simulink model "simulator"  (R2019b)
settings: Solver=ode3  StartTime=0.0  StopTime=inf  FixedStep=0.5  RelTol=1e-3
InitFcn:
  | load('sim_buses');
undefined symbols (not defined in the file or in its folder): m, n
settings Model: OrderedModelArguments=off  Creator=Rafael.Casado  LastModifiedBy=paloma

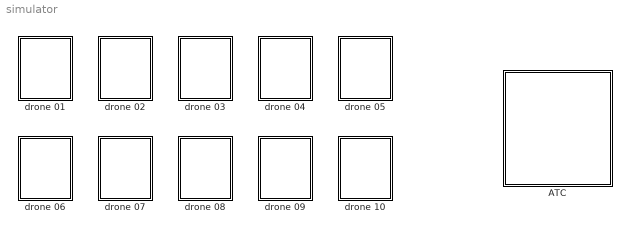
== system simulator ==
  ATC : Subsystem
      mask Display: image('$imagefile'); % Use "Edit Image" on toolstrip to change.
  drone 01 : Subsystem
      mask Display:
      | patch([50 -50 -50 50], [40 40 -60 -60], [1 1 1])
      | 
      | patch([8 -8 -8 8], [6 6 -6 -6], [0.7 0.7 0.7])
      | 
      | patch([ 8  8  28  28], [2 0 0 2], [0.5 0.5 0.5])
      | patch([-8 -8 -28 -28], [2 0 0 2], [0.5 0.5 0.5])
      | 
      | patch([ 30  46  30  14], [6 5 4 5], [1 0 0])
      | patch([-30 -46 -30 -14], [6 5 4 5], [1 0 0])
      | 
      | patch([ 28  28  32  32], [4 -2 -2 4], [0 0 0])
      | patch([-28 -28 -32 -32], [4 -2 -2 4], [0 0 0])
      | 
      | patch([ 8  12  11  7], [-6 -18 -18 -6], [0 0 0])
      | patch([-8 -12 -11 -7], [-6 -18 -18 -6], [0 0 0])
  drone 02 : Subsystem
      mask Display:
      | patch([50 -50 -50 50], [40 40 -60 -60], [1 1 1])
      | 
      | patch([8 -8 -8 8], [6 6 -6 -6], [0.7 0.7 0.7])
      | 
      | patch([ 8  8  28  28], [2 0 0 2], [0.5 0.5 0.5])
      | patch([-8 -8 -28 -28], [2 0 0 2], [0.5 0.5 0.5])
      | 
      | patch([ 30  46  30  14], [6 5 4 5], [1 0 0])
      | patch([-30 -46 -30 -14], [6 5 4 5], [1 0 0])
      | 
      | patch([ 28  28  32  32], [4 -2 -2 4], [0 0 0])
      | patch([-28 -28 -32 -32], [4 -2 -2 4], [0 0 0])
      | 
      | patch([ 8  12  11  7], [-6 -18 -18 -6], [0 0 0])
      | patch([-8 -12 -11 -7], [-6 -18 -18 -6], [0 0 0])
  drone 03 : Subsystem
      mask Display:
      | patch([50 -50 -50 50], [40 40 -60 -60], [1 1 1])
      | 
      | patch([8 -8 -8 8], [6 6 -6 -6], [0.7 0.7 0.7])
      | 
      | patch([ 8  8  28  28], [2 0 0 2], [0.5 0.5 0.5])
      | patch([-8 -8 -28 -28], [2 0 0 2], [0.5 0.5 0.5])
      | 
      | patch([ 30  46  30  14], [6 5 4 5], [1 0 0])
      | patch([-30 -46 -30 -14], [6 5 4 5], [1 0 0])
      | 
      | patch([ 28  28  32  32], [4 -2 -2 4], [0 0 0])
      | patch([-28 -28 -32 -32], [4 -2 -2 4], [0 0 0])
      | 
      | patch([ 8  12  11  7], [-6 -18 -18 -6], [0 0 0])
      | patch([-8 -12 -11 -7], [-6 -18 -18 -6], [0 0 0])
  drone 04 : Subsystem
      mask Display:
      | patch([50 -50 -50 50], [40 40 -60 -60], [1 1 1])
      | 
      | patch([8 -8 -8 8], [6 6 -6 -6], [0.7 0.7 0.7])
      | 
      | patch([ 8  8  28  28], [2 0 0 2], [0.5 0.5 0.5])
      | patch([-8 -8 -28 -28], [2 0 0 2], [0.5 0.5 0.5])
      | 
      | patch([ 30  46  30  14], [6 5 4 5], [1 0 0])
      | patch([-30 -46 -30 -14], [6 5 4 5], [1 0 0])
      | 
      | patch([ 28  28  32  32], [4 -2 -2 4], [0 0 0])
      | patch([-28 -28 -32 -32], [4 -2 -2 4], [0 0 0])
      | 
      | patch([ 8  12  11  7], [-6 -18 -18 -6], [0 0 0])
      | patch([-8 -12 -11 -7], [-6 -18 -18 -6], [0 0 0])
  drone 05 : Subsystem
      mask Display:
      | patch([50 -50 -50 50], [40 40 -60 -60], [1 1 1])
      | 
      | patch([8 -8 -8 8], [6 6 -6 -6], [0.7 0.7 0.7])
      | 
      | patch([ 8  8  28  28], [2 0 0 2], [0.5 0.5 0.5])
      | patch([-8 -8 -28 -28], [2 0 0 2], [0.5 0.5 0.5])
      | 
      | patch([ 30  46  30  14], [6 5 4 5], [1 0 0])
      | patch([-30 -46 -30 -14], [6 5 4 5], [1 0 0])
      | 
      | patch([ 28  28  32  32], [4 -2 -2 4], [0 0 0])
      | patch([-28 -28 -32 -32], [4 -2 -2 4], [0 0 0])
      | 
      | patch([ 8  12  11  7], [-6 -18 -18 -6], [0 0 0])
      | patch([-8 -12 -11 -7], [-6 -18 -18 -6], [0 0 0])
  drone 06 : Subsystem
      mask Display:
      | patch([50 -50 -50 50], [40 40 -60 -60], [1 1 1])
      | 
      | patch([8 -8 -8 8], [6 6 -6 -6], [0.7 0.7 0.7])
      | 
      | patch([ 8  8  28  28], [2 0 0 2], [0.5 0.5 0.5])
      | patch([-8 -8 -28 -28], [2 0 0 2], [0.5 0.5 0.5])
      | 
      | patch([ 30  46  30  14], [6 5 4 5], [1 0 0])
      | patch([-30 -46 -30 -14], [6 5 4 5], [1 0 0])
      | 
      | patch([ 28  28  32  32], [4 -2 -2 4], [0 0 0])
      | patch([-28 -28 -32 -32], [4 -2 -2 4], [0 0 0])
      | 
      | patch([ 8  12  11  7], [-6 -18 -18 -6], [0 0 0])
      | patch([-8 -12 -11 -7], [-6 -18 -18 -6], [0 0 0])
  drone 07 : Subsystem
      mask Display:
      | patch([50 -50 -50 50], [40 40 -60 -60], [1 1 1])
      | 
      | patch([8 -8 -8 8], [6 6 -6 -6], [0.7 0.7 0.7])
      | 
      | patch([ 8  8  28  28], [2 0 0 2], [0.5 0.5 0.5])
      | patch([-8 -8 -28 -28], [2 0 0 2], [0.5 0.5 0.5])
      | 
      | patch([ 30  46  30  14], [6 5 4 5], [1 0 0])
      | patch([-30 -46 -30 -14], [6 5 4 5], [1 0 0])
      | 
      | patch([ 28  28  32  32], [4 -2 -2 4], [0 0 0])
      | patch([-28 -28 -32 -32], [4 -2 -2 4], [0 0 0])
      | 
      | patch([ 8  12  11  7], [-6 -18 -18 -6], [0 0 0])
      | patch([-8 -12 -11 -7], [-6 -18 -18 -6], [0 0 0])
  drone 08 : Subsystem
      mask Display:
      | patch([50 -50 -50 50], [40 40 -60 -60], [1 1 1])
      | 
      | patch([8 -8 -8 8], [6 6 -6 -6], [0.7 0.7 0.7])
      | 
      | patch([ 8  8  28  28], [2 0 0 2], [0.5 0.5 0.5])
      | patch([-8 -8 -28 -28], [2 0 0 2], [0.5 0.5 0.5])
      | 
      | patch([ 30  46  30  14], [6 5 4 5], [1 0 0])
      | patch([-30 -46 -30 -14], [6 5 4 5], [1 0 0])
      | 
      | patch([ 28  28  32  32], [4 -2 -2 4], [0 0 0])
      | patch([-28 -28 -32 -32], [4 -2 -2 4], [0 0 0])
      | 
      | patch([ 8  12  11  7], [-6 -18 -18 -6], [0 0 0])
      | patch([-8 -12 -11 -7], [-6 -18 -18 -6], [0 0 0])
  drone 09 : Subsystem
      mask Display:
      | patch([50 -50 -50 50], [40 40 -60 -60], [1 1 1])
      | 
      | patch([8 -8 -8 8], [6 6 -6 -6], [0.7 0.7 0.7])
      | 
      | patch([ 8  8  28  28], [2 0 0 2], [0.5 0.5 0.5])
      | patch([-8 -8 -28 -28], [2 0 0 2], [0.5 0.5 0.5])
      | 
      | patch([ 30  46  30  14], [6 5 4 5], [1 0 0])
      | patch([-30 -46 -30 -14], [6 5 4 5], [1 0 0])
      | 
      | patch([ 28  28  32  32], [4 -2 -2 4], [0 0 0])
      | patch([-28 -28 -32 -32], [4 -2 -2 4], [0 0 0])
      | 
      | patch([ 8  12  11  7], [-6 -18 -18 -6], [0 0 0])
      | patch([-8 -12 -11 -7], [-6 -18 -18 -6], [0 0 0])
  drone 10 : Subsystem
      mask Display:
      | patch([50 -50 -50 50], [40 40 -60 -60], [1 1 1])
      | 
      | patch([8 -8 -8 8], [6 6 -6 -6], [0.7 0.7 0.7])
      | 
      | patch([ 8  8  28  28], [2 0 0 2], [0.5 0.5 0.5])
      | patch([-8 -8 -28 -28], [2 0 0 2], [0.5 0.5 0.5])
      | 
      | patch([ 30  46  30  14], [6 5 4 5], [1 0 0])
      | patch([-30 -46 -30 -14], [6 5 4 5], [1 0 0])
      | 
      | patch([ 28  28  32  32], [4 -2 -2 4], [0 0 0])
      | patch([-28 -28 -32 -32], [4 -2 -2 4], [0 0 0])
      | 
      | patch([ 8  12  11  7], [-6 -18 -18 -6], [0 0 0])
      | patch([-8 -12 -11 -7], [-6 -18 -18 -6], [0 0 0])

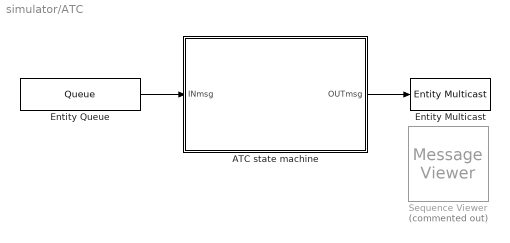
== system simulator/ATC ==
  ATC state machine : Stateflow chart  TreatAsAtomicUnit=on
  Entity Multicast : EntityMulticast  InputPortMessageModes=m  MulticastTag=msg
  Entity Queue : Queue  OutputPortMessageModes=m  Capacity=200  EntityArrivalSource=Multicast  MulticastTag=msg
  Sequence Viewer : MessageViewer  Commented=on  History=1000
  wires:
  Entity Queue/1 -> ATC state machine/1(INmsg)
  ATC state machine/1(OUTmsg) -> Entity Multicast/1

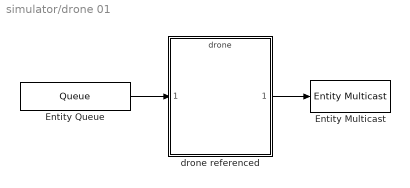
== system simulator/drone 01 ==
  Entity Multicast : EntityMulticast  InputPortMessageModes=m  MulticastTag=msg
  Entity Queue : Queue  OutputPortMessageModes=m  Capacity=105  EntityArrivalSource=Multicast  MulticastTag=msg
  drone referenced : ModelReference  InputPortMessageModes=m  OutputPortMessageModes=m  ModelNameDialog=drone  ParameterArgumentNames=UAVid  ParameterArgumentValues=1  UsingDefaultArgumentValue=0  SimulationMode=Normal  ModelReferenceVersion=1.1019
      mask Display:
      | patch([50 -50 -50 50], [40 40 -60 -60], [1 1 1])
      | 
      | patch([8 -8 -8 8], [6 6 -6 -6], [0.7 0.7 0.7])
      | 
      | patch([ 8  8  28  28], [2 0 0 2], [0.5 0.5 0.5])
      | patch([-8 -8 -28 -28], [2 0 0 2], [0.5 0.5 0.5])
      | 
      | patch([ 30  46  30  14], [6 5 4 5], [1 0 0])
      | patch([-30 -46 -30 -14], [6 5 4 5], [1 0 0])
      | 
      | patch([ 28  28  32  32], [4 -2 -2 4], [0 0 0])
      | patch([-28 -28 -32 -32], [4 -2 -2 4], [0 0 0])
      | 
      | patch([ 8  12  11  7], [-6 -18 -18 -6], [0 0 0])
      | patch([-8 -12 -11 -7], [-6 -18 -18 -6], [0 0 0])
  wires:
  drone referenced/1 -> Entity Multicast/1
  Entity Queue/1 -> drone referenced/1

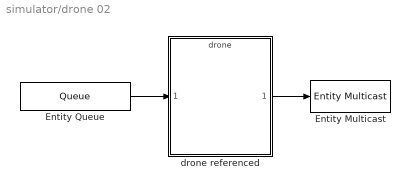
== system simulator/drone 02 ==
  Entity Multicast : EntityMulticast  InputPortMessageModes=m  MulticastTag=msg
  Entity Queue : Queue  OutputPortMessageModes=m  Capacity=105  EntityArrivalSource=Multicast  MulticastTag=msg
  drone referenced : ModelReference  InputPortMessageModes=m  OutputPortMessageModes=m  ModelNameDialog=drone  ParameterArgumentNames=UAVid  ParameterArgumentValues=2  UsingDefaultArgumentValue=0  SimulationMode=Normal  ModelReferenceVersion=1.1019
      mask Display:
      | patch([50 -50 -50 50], [40 40 -60 -60], [1 1 1])
      | 
      | patch([8 -8 -8 8], [6 6 -6 -6], [0.7 0.7 0.7])
      | 
      | patch([ 8  8  28  28], [2 0 0 2], [0.5 0.5 0.5])
      | patch([-8 -8 -28 -28], [2 0 0 2], [0.5 0.5 0.5])
      | 
      | patch([ 30  46  30  14], [6 5 4 5], [1 0 0])
      | patch([-30 -46 -30 -14], [6 5 4 5], [1 0 0])
      | 
      | patch([ 28  28  32  32], [4 -2 -2 4], [0 0 0])
      | patch([-28 -28 -32 -32], [4 -2 -2 4], [0 0 0])
      | 
      | patch([ 8  12  11  7], [-6 -18 -18 -6], [0 0 0])
      | patch([-8 -12 -11 -7], [-6 -18 -18 -6], [0 0 0])
  wires:
  drone referenced/1 -> Entity Multicast/1
  Entity Queue/1 -> drone referenced/1

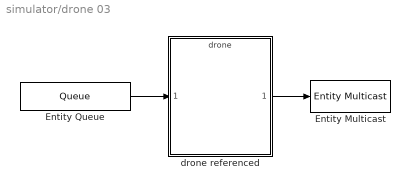
== system simulator/drone 03 ==
  Entity Multicast : EntityMulticast  InputPortMessageModes=m  MulticastTag=msg
  Entity Queue : Queue  OutputPortMessageModes=m  Capacity=105  EntityArrivalSource=Multicast  MulticastTag=msg
  drone referenced : ModelReference  InputPortMessageModes=m  OutputPortMessageModes=m  ModelNameDialog=drone  ParameterArgumentNames=UAVid  ParameterArgumentValues=3  UsingDefaultArgumentValue=0  SimulationMode=Normal  ModelReferenceVersion=1.1019
      mask Display:
      | patch([50 -50 -50 50], [40 40 -60 -60], [1 1 1])
      | 
      | patch([8 -8 -8 8], [6 6 -6 -6], [0.7 0.7 0.7])
      | 
      | patch([ 8  8  28  28], [2 0 0 2], [0.5 0.5 0.5])
      | patch([-8 -8 -28 -28], [2 0 0 2], [0.5 0.5 0.5])
      | 
      | patch([ 30  46  30  14], [6 5 4 5], [1 0 0])
      | patch([-30 -46 -30 -14], [6 5 4 5], [1 0 0])
      | 
      | patch([ 28  28  32  32], [4 -2 -2 4], [0 0 0])
      | patch([-28 -28 -32 -32], [4 -2 -2 4], [0 0 0])
      | 
      | patch([ 8  12  11  7], [-6 -18 -18 -6], [0 0 0])
      | patch([-8 -12 -11 -7], [-6 -18 -18 -6], [0 0 0])
  wires:
  drone referenced/1 -> Entity Multicast/1
  Entity Queue/1 -> drone referenced/1

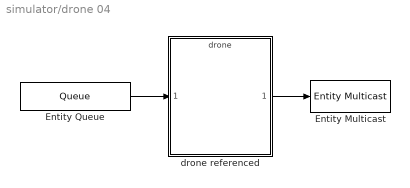
== system simulator/drone 04 ==
  Entity Multicast : EntityMulticast  InputPortMessageModes=m  MulticastTag=msg
  Entity Queue : Queue  OutputPortMessageModes=m  Capacity=105  EntityArrivalSource=Multicast  MulticastTag=msg
  drone referenced : ModelReference  InputPortMessageModes=m  OutputPortMessageModes=m  ModelNameDialog=drone  ParameterArgumentNames=UAVid  ParameterArgumentValues=4  UsingDefaultArgumentValue=0  SimulationMode=Normal  ModelReferenceVersion=1.1019
      mask Display:
      | patch([50 -50 -50 50], [40 40 -60 -60], [1 1 1])
      | 
      | patch([8 -8 -8 8], [6 6 -6 -6], [0.7 0.7 0.7])
      | 
      | patch([ 8  8  28  28], [2 0 0 2], [0.5 0.5 0.5])
      | patch([-8 -8 -28 -28], [2 0 0 2], [0.5 0.5 0.5])
      | 
      | patch([ 30  46  30  14], [6 5 4 5], [1 0 0])
      | patch([-30 -46 -30 -14], [6 5 4 5], [1 0 0])
      | 
      | patch([ 28  28  32  32], [4 -2 -2 4], [0 0 0])
      | patch([-28 -28 -32 -32], [4 -2 -2 4], [0 0 0])
      | 
      | patch([ 8  12  11  7], [-6 -18 -18 -6], [0 0 0])
      | patch([-8 -12 -11 -7], [-6 -18 -18 -6], [0 0 0])
  wires:
  drone referenced/1 -> Entity Multicast/1
  Entity Queue/1 -> drone referenced/1

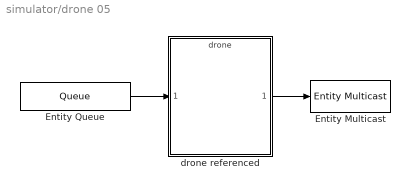
== system simulator/drone 05 ==
  Entity Multicast : EntityMulticast  InputPortMessageModes=m  MulticastTag=msg
  Entity Queue : Queue  OutputPortMessageModes=m  Capacity=105  EntityArrivalSource=Multicast  MulticastTag=msg
  drone referenced : ModelReference  InputPortMessageModes=m  OutputPortMessageModes=m  ModelNameDialog=drone  ParameterArgumentNames=UAVid  ParameterArgumentValues=5  UsingDefaultArgumentValue=0  SimulationMode=Normal  ModelReferenceVersion=1.1019
      mask Display:
      | patch([50 -50 -50 50], [40 40 -60 -60], [1 1 1])
      | 
      | patch([8 -8 -8 8], [6 6 -6 -6], [0.7 0.7 0.7])
      | 
      | patch([ 8  8  28  28], [2 0 0 2], [0.5 0.5 0.5])
      | patch([-8 -8 -28 -28], [2 0 0 2], [0.5 0.5 0.5])
      | 
      | patch([ 30  46  30  14], [6 5 4 5], [1 0 0])
      | patch([-30 -46 -30 -14], [6 5 4 5], [1 0 0])
      | 
      | patch([ 28  28  32  32], [4 -2 -2 4], [0 0 0])
      | patch([-28 -28 -32 -32], [4 -2 -2 4], [0 0 0])
      | 
      | patch([ 8  12  11  7], [-6 -18 -18 -6], [0 0 0])
      | patch([-8 -12 -11 -7], [-6 -18 -18 -6], [0 0 0])
  wires:
  drone referenced/1 -> Entity Multicast/1
  Entity Queue/1 -> drone referenced/1

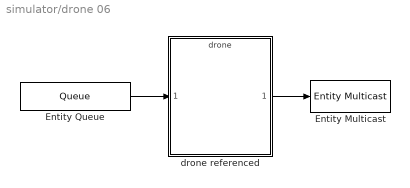
== system simulator/drone 06 ==
  Entity Multicast : EntityMulticast  InputPortMessageModes=m  MulticastTag=msg
  Entity Queue : Queue  OutputPortMessageModes=m  Capacity=105  EntityArrivalSource=Multicast  MulticastTag=msg
  drone referenced : ModelReference  InputPortMessageModes=m  OutputPortMessageModes=m  ModelNameDialog=drone  ParameterArgumentNames=UAVid  ParameterArgumentValues=6  UsingDefaultArgumentValue=0  SimulationMode=Normal  ModelReferenceVersion=1.1019
      mask Display:
      | patch([50 -50 -50 50], [40 40 -60 -60], [1 1 1])
      | 
      | patch([8 -8 -8 8], [6 6 -6 -6], [0.7 0.7 0.7])
      | 
      | patch([ 8  8  28  28], [2 0 0 2], [0.5 0.5 0.5])
      | patch([-8 -8 -28 -28], [2 0 0 2], [0.5 0.5 0.5])
      | 
      | patch([ 30  46  30  14], [6 5 4 5], [1 0 0])
      | patch([-30 -46 -30 -14], [6 5 4 5], [1 0 0])
      | 
      | patch([ 28  28  32  32], [4 -2 -2 4], [0 0 0])
      | patch([-28 -28 -32 -32], [4 -2 -2 4], [0 0 0])
      | 
      | patch([ 8  12  11  7], [-6 -18 -18 -6], [0 0 0])
      | patch([-8 -12 -11 -7], [-6 -18 -18 -6], [0 0 0])
  wires:
  drone referenced/1 -> Entity Multicast/1
  Entity Queue/1 -> drone referenced/1

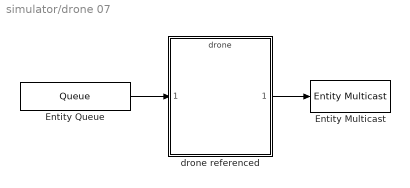
== system simulator/drone 07 ==
  Entity Multicast : EntityMulticast  InputPortMessageModes=m  MulticastTag=msg
  Entity Queue : Queue  OutputPortMessageModes=m  Capacity=105  EntityArrivalSource=Multicast  MulticastTag=msg
  drone referenced : ModelReference  InputPortMessageModes=m  OutputPortMessageModes=m  ModelNameDialog=drone  ParameterArgumentNames=UAVid  ParameterArgumentValues=7  UsingDefaultArgumentValue=0  SimulationMode=Normal  ModelReferenceVersion=1.1019
      mask Display:
      | patch([50 -50 -50 50], [40 40 -60 -60], [1 1 1])
      | 
      | patch([8 -8 -8 8], [6 6 -6 -6], [0.7 0.7 0.7])
      | 
      | patch([ 8  8  28  28], [2 0 0 2], [0.5 0.5 0.5])
      | patch([-8 -8 -28 -28], [2 0 0 2], [0.5 0.5 0.5])
      | 
      | patch([ 30  46  30  14], [6 5 4 5], [1 0 0])
      | patch([-30 -46 -30 -14], [6 5 4 5], [1 0 0])
      | 
      | patch([ 28  28  32  32], [4 -2 -2 4], [0 0 0])
      | patch([-28 -28 -32 -32], [4 -2 -2 4], [0 0 0])
      | 
      | patch([ 8  12  11  7], [-6 -18 -18 -6], [0 0 0])
      | patch([-8 -12 -11 -7], [-6 -18 -18 -6], [0 0 0])
  wires:
  drone referenced/1 -> Entity Multicast/1
  Entity Queue/1 -> drone referenced/1

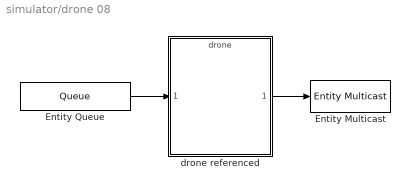
== system simulator/drone 08 ==
  Entity Multicast : EntityMulticast  InputPortMessageModes=m  MulticastTag=msg
  Entity Queue : Queue  OutputPortMessageModes=m  Capacity=105  EntityArrivalSource=Multicast  MulticastTag=msg
  drone referenced : ModelReference  InputPortMessageModes=m  OutputPortMessageModes=m  ModelNameDialog=drone  ParameterArgumentNames=UAVid  ParameterArgumentValues=8  UsingDefaultArgumentValue=0  SimulationMode=Normal  ModelReferenceVersion=1.1019
      mask Display:
      | patch([50 -50 -50 50], [40 40 -60 -60], [1 1 1])
      | 
      | patch([8 -8 -8 8], [6 6 -6 -6], [0.7 0.7 0.7])
      | 
      | patch([ 8  8  28  28], [2 0 0 2], [0.5 0.5 0.5])
      | patch([-8 -8 -28 -28], [2 0 0 2], [0.5 0.5 0.5])
      | 
      | patch([ 30  46  30  14], [6 5 4 5], [1 0 0])
      | patch([-30 -46 -30 -14], [6 5 4 5], [1 0 0])
      | 
      | patch([ 28  28  32  32], [4 -2 -2 4], [0 0 0])
      | patch([-28 -28 -32 -32], [4 -2 -2 4], [0 0 0])
      | 
      | patch([ 8  12  11  7], [-6 -18 -18 -6], [0 0 0])
      | patch([-8 -12 -11 -7], [-6 -18 -18 -6], [0 0 0])
  wires:
  drone referenced/1 -> Entity Multicast/1
  Entity Queue/1 -> drone referenced/1

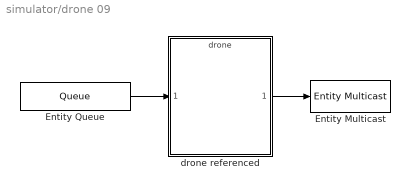
== system simulator/drone 09 ==
  Entity Multicast : EntityMulticast  InputPortMessageModes=m  MulticastTag=msg
  Entity Queue : Queue  OutputPortMessageModes=m  Capacity=105  EntityArrivalSource=Multicast  MulticastTag=msg
  drone referenced : ModelReference  InputPortMessageModes=m  OutputPortMessageModes=m  ModelNameDialog=drone  ParameterArgumentNames=UAVid  ParameterArgumentValues=9  UsingDefaultArgumentValue=0  SimulationMode=Normal  ModelReferenceVersion=1.1019
      mask Display:
      | patch([50 -50 -50 50], [40 40 -60 -60], [1 1 1])
      | 
      | patch([8 -8 -8 8], [6 6 -6 -6], [0.7 0.7 0.7])
      | 
      | patch([ 8  8  28  28], [2 0 0 2], [0.5 0.5 0.5])
      | patch([-8 -8 -28 -28], [2 0 0 2], [0.5 0.5 0.5])
      | 
      | patch([ 30  46  30  14], [6 5 4 5], [1 0 0])
      | patch([-30 -46 -30 -14], [6 5 4 5], [1 0 0])
      | 
      | patch([ 28  28  32  32], [4 -2 -2 4], [0 0 0])
      | patch([-28 -28 -32 -32], [4 -2 -2 4], [0 0 0])
      | 
      | patch([ 8  12  11  7], [-6 -18 -18 -6], [0 0 0])
      | patch([-8 -12 -11 -7], [-6 -18 -18 -6], [0 0 0])
  wires:
  drone referenced/1 -> Entity Multicast/1
  Entity Queue/1 -> drone referenced/1

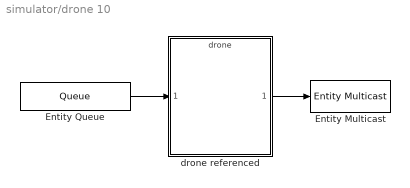
== system simulator/drone 10 ==
  Entity Multicast : EntityMulticast  InputPortMessageModes=m  MulticastTag=msg
  Entity Queue : Queue  OutputPortMessageModes=m  Capacity=105  EntityArrivalSource=Multicast  MulticastTag=msg
  drone referenced : ModelReference  InputPortMessageModes=m  OutputPortMessageModes=m  ModelNameDialog=drone  ParameterArgumentNames=UAVid  ParameterArgumentValues=10  UsingDefaultArgumentValue=0  SimulationMode=Normal  ModelReferenceVersion=1.1019
      mask Display:
      | patch([50 -50 -50 50], [40 40 -60 -60], [1 1 1])
      | 
      | patch([8 -8 -8 8], [6 6 -6 -6], [0.7 0.7 0.7])
      | 
      | patch([ 8  8  28  28], [2 0 0 2], [0.5 0.5 0.5])
      | patch([-8 -8 -28 -28], [2 0 0 2], [0.5 0.5 0.5])
      | 
      | patch([ 30  46  30  14], [6 5 4 5], [1 0 0])
      | patch([-30 -46 -30 -14], [6 5 4 5], [1 0 0])
      | 
      | patch([ 28  28  32  32], [4 -2 -2 4], [0 0 0])
      | patch([-28 -28 -32 -32], [4 -2 -2 4], [0 0 0])
      | 
      | patch([ 8  12  11  7], [-6 -18 -18 -6], [0 0 0])
      | patch([-8 -12 -11 -7], [-6 -18 -18 -6], [0 0 0])
  wires:
  drone referenced/1 -> Entity Multicast/1
  Entity Queue/1 -> drone referenced/1

== stateflow chart simulator/ATC/ATC state machine ==
  state CONTROL
    msgsProcess
    state msgsProcess [function]
      (default) -> (junction 50)
      (junction 50) -> (junction 49) [order 1] : INmsg
      (junction 48) -> (junction 50)
      (junction 50) -> (junction 53) [order 2]
      (junction 49) -> (junction 48) : {ATMmsgProcess}
  (default) -> CONTROL
  data: INmsg input Bus: bus_msg; OUTmsg output Bus: bus_msg; ATClist local Bus: ATCrecord size=50; numUAVs local =0
  function ATMmsgProcess:
    | function ATMmsgProcess
    | coder.extrinsic('get_param','set_param','evalin')
    | 
    | % Inicialización de ATC
    | persistent numUAVs logDelivery packages outputLog
    | 
    | 
    | if(isempty(logDelivery))
    | 
    |     %Fichero de posiciones de entrega
    |     logDelivery = fopen('logDelivery.csv','w');
    |     
    |     %Fichero log de salida
    |     outputLog = fopen('outputLog.csv','w');
    |     
    |     % Leo posiciones iniciales (*appDesigner)
    |     initPos = evalin('base','initPos');
    |     numUAVs = length(initPos);
    |     
    |      for i = 1:numUAVs
    |          ATClist(i).UAVid     = i;
    |          ATClist(i).available = false;
    |          ATClist(i).home      = false;
    |          ATClist(i).end       = false;
    |          ATClist(i).px_init   = initPos(i,1);
    |          ATClist(i).py_init   = initPos(i,2);
    |          
    |         % Inserto registro en log 'outputLog' (código 01: posiciones iniciales UAV)
    |          fprintf(outputLog,"01,%03.0f,%+05.2f,%05.2f\n" ...
    |              ,ATClist(i).UAVid       ...
    |              ,ATClist(i).px_init     ...
    |              ,ATClist(i).py_init);
    |      end
    |          
    |     % Leo matriz entrega de paquetes (*appDesigner)
    |     packages = evalin('base','packages');
    | 
    | end
    | 
    | %Fichero log de salida
    | outputLog = fopen('outputLog.csv','a');
    | 
    | % extraigo informacion del mensaje
    | msg   = INmsg.data;
    | UAVid = msg.id; 
    | discard(INmsg)
    | 
    | % descarto eco de mensajes propios
    | if msg.senderATC  
    |    return
    | end
    | 
    | curTime = get_param('simulator','SimulationTime');
    | 
    | if msg.available && ~ATClist(UAVid).available
    | % el drone esta disponible para nueva orden
    | 
    |     if ATClist(UAVid).home
    |         % el drone ha retornado a casa
    |         
    |         % Inserto registro en log 'outputLog' (código 04: UAV ha llegado a casa)
    |         fprintf(outputLog,"04,%05.0f,%03.0f\n" ...
    |                  ,curTime           ...
    |                  ,UAVid);
    |                  
    |         ATClist(UAVid).end = true;
    |         fprintf('%6.1f: Drone %.0f ha regresado\n',curTime,UAVid);
    | 
    |         % Compruebo si todos han terminado
    |         todosEnCasa = true;
    |         for i = 1:numUAVs
    |             if ~ATClist(i).end
    |                 todosEnCasa = false;
    |                 break
    |             end
    |         end
    |         if todosEnCasa
    |             fprintf('%6.1f: Todos los drones han regresado\n',curTime);
    |             % Inserto registro en log 'outputLog' (código 05: Todos los drones han regresado)
    |             fprintf(outputLog,"05,%05.0f\n" ...
    |                  ,curTime);
    |             set_param('simulator', 'SimulationCommand', 'stop');
    |         end 
    |         
    |     else
    |         % el drone aun tiene que viajar
    |         OUTmsg.data.id        = UAVid;
    |         OUTmsg.data.senderATC = true;
    |         OUTmsg.data.z         = 0;
    |         OUTmsg.data.vx        = 0;
    |         OUTmsg.data.vy        = 0;
    |         OUTmsg.data.vz        = 0;
    | 
    |         if ~isempty(packages)
    | 
    |             % ordeno entrega de paquete
    |             OUTmsg.data.x = packages(1,1);
    |             OUTmsg.data.y = packages(1,2);
    |             fprintf('%6.1f: ATC ordena nueva entrega a drone %.0f\n',curTime,UAVid);
    |             
    |             % Inserto registro en log 'outputLog' (código 02: orden de paquete)
    |             fprintf(outputLog,"02,%05.0f,%03.0f,%+05.2f,%05.2f\n" ...
    |                      ,curTime           ...
    |                      ,UAVid             ...
    |                      ,OUTmsg.data.x     ...
    |                      ,OUTmsg.data.y);
    | 
    |             %Elimino paquete de la lista de entrega
    |             l = double(0);
    |             l = size(packages,1);
    |             if l > 1
    |                 packages = packages(2:l,1:2);
    |             else
    |                 packages = [];
    |             end
    | 
    |         else
    |             % envio al drone a casa
    |             ATClist(UAVid).home = true;
    |             OUTmsg.data.x = ATClist(UAVid).px_init;
    |             OUTmsg.data.y = ATClist(UAVid).py_init;
    |             fprintf('%6.1f: ATC ordena a drone %.0f regresar a casa\n',curTime,UAVid);
    |             
    |             % Inserto registro en log 'outputLog' (código 03: orden vuelta a casa UAV)
    |             fprintf(outputLog,"03,%05.0f,%03.0f\n" ...
    |                      ,curTime           ...
    |                      ,UAVid);
    |         end
    | 
    |         send(OUTmsg);
    | 
    |         % Inserto registro en log 'logDelivery'
    |         fprintf(logDelivery,"%05.0f,%03.0f,%+05.2f,%05.2f\n" ...
    |                      ,curTime           ...
    |                      ,UAVid             ...
    |                      ,OUTmsg.data.x     ...
    |                      ,OUTmsg.data.y);  
    |         
    | 
    |     end
    | 
    | end
    | 
    | % actualizo situación de disponibilidad
    | % es importante primero comprobar y luego actualizar, para que funcione
    | % correctamente solo la primera vez que se recibe el mensaje
    | ATClist(msg.id).available = msg.available;
    | 
    | % cierro fichero Log
    | fclose(outputLog);
